simulink model "HealthySubject08062023_Storage"  (R2023a)
settings: Solver=VariableStepAuto  StartTime=0.0  StopTime=3000  RelTol=1e-3
values from neighbouring files (symbols this model uses):
  Cn = 1    [Inhibitory_excitatory_ULInjury_1Hz_08102023.m]    (also in Inhibitory_excitatory_ULInjury_30Hz_08102023.m; InitialExcitatoryInhibitoryNeurons_Healthy08062023.m; InitialExcitatoryInhibitoryULInjured_08102023_DSD.m)
  EK = -84*1    (= -84)    [Inhibitory_excitatory_ULInjury_1Hz_08102023.m]    (also in Inhibitory_excitatory_ULInjury_30Hz_08102023.m; InitialExcitatoryInhibitoryNeurons_Healthy08062023.m; InitialExcitatoryInhibitoryULInjured_08102023_DSD.m)
  EKEx = -90    [Inhibitory_excitatory_ULInjury_1Hz_08102023.m]    (also in Inhibitory_excitatory_ULInjury_30Hz_08102023.m; InitialExcitatoryInhibitoryNeurons_Healthy08062023.m; InitialExcitatoryInhibitoryULInjured_08102023_DSD.m)
  EKIn = -90    [Inhibitory_excitatory_ULInjury_1Hz_08102023.m]    (also in Inhibitory_excitatory_ULInjury_30Hz_08102023.m; InitialExcitatoryInhibitoryNeurons_Healthy08062023.m; InitialExcitatoryInhibitoryULInjured_08102023_DSD.m)
  ELEx = -65    [Inhibitory_excitatory_ULInjury_1Hz_08102023.m]    (also in Inhibitory_excitatory_ULInjury_30Hz_08102023.m; InitialExcitatoryInhibitoryNeurons_Healthy08062023.m; InitialExcitatoryInhibitoryULInjured_08102023_DSD.m)
  ELIn = -65    [Inhibitory_excitatory_ULInjury_1Hz_08102023.m]    (also in Inhibitory_excitatory_ULInjury_30Hz_08102023.m; InitialExcitatoryInhibitoryNeurons_Healthy08062023.m; InitialExcitatoryInhibitoryULInjured_08102023_DSD.m)
  ELk = -83.38*1    (= -83.38)    [Inhibitory_excitatory_ULInjury_1Hz_08102023.m]    (also in Inhibitory_excitatory_ULInjury_30Hz_08102023.m; InitialExcitatoryInhibitoryNeurons_Healthy08062023.m; InitialExcitatoryInhibitoryULInjured_08102023_DSD.m)
  ENa = 50*1    (= 50)    [Inhibitory_excitatory_ULInjury_1Hz_08102023.m]    (also in Inhibitory_excitatory_ULInjury_30Hz_08102023.m; InitialExcitatoryInhibitoryNeurons_Healthy08062023.m; InitialExcitatoryInhibitoryULInjured_08102023_DSD.m)
  ENaEx = 60    [Inhibitory_excitatory_ULInjury_1Hz_08102023.m]    (also in Inhibitory_excitatory_ULInjury_30Hz_08102023.m; InitialExcitatoryInhibitoryNeurons_Healthy08062023.m; InitialExcitatoryInhibitoryULInjured_08102023_DSD.m)
  ENaIn = 55    [Inhibitory_excitatory_ULInjury_1Hz_08102023.m]    (also in Inhibitory_excitatory_ULInjury_30Hz_08102023.m; InitialExcitatoryInhibitoryNeurons_Healthy08062023.m; InitialExcitatoryInhibitoryULInjured_08102023_DSD.m)
  ErestE = -65    [Inhibitory_excitatory_ULInjury_1Hz_08102023.m]    (also in Inhibitory_excitatory_ULInjury_30Hz_08102023.m; InitialExcitatoryInhibitoryNeurons_Healthy08062023.m; InitialExcitatoryInhibitoryULInjured_08102023_DSD.m)
  ErestIn = -64    [Inhibitory_excitatory_ULInjury_1Hz_08102023.m]    (also in Inhibitory_excitatory_ULInjury_30Hz_08102023.m; InitialExcitatoryInhibitoryNeurons_Healthy08062023.m; InitialExcitatoryInhibitoryULInjured_08102023_DSD.m)
  ESynE = -10    [Inhibitory_excitatory_ULInjury_1Hz_08102023.m]    (also in Inhibitory_excitatory_ULInjury_30Hz_08102023.m; InitialExcitatoryInhibitoryNeurons_Healthy08062023.m; InitialExcitatoryInhibitoryULInjured_08102023_DSD.m)
  ESynE2 = -10    [Inhibitory_excitatory_ULInjury_1Hz_08102023.m]    (also in Inhibitory_excitatory_ULInjury_30Hz_08102023.m; InitialExcitatoryInhibitoryNeurons_Healthy08062023.m; InitialExcitatoryInhibitoryULInjured_08102023_DSD.m)
  ESynE3 = -10    [Inhibitory_excitatory_ULInjury_1Hz_08102023.m]    (also in Inhibitory_excitatory_ULInjury_30Hz_08102023.m; InitialExcitatoryInhibitoryNeurons_Healthy08062023.m; InitialExcitatoryInhibitoryULInjured_08102023_DSD.m)
  ESynE4 = -10    [Inhibitory_excitatory_ULInjury_1Hz_08102023.m]    (also in Inhibitory_excitatory_ULInjury_30Hz_08102023.m; InitialExcitatoryInhibitoryNeurons_Healthy08062023.m; InitialExcitatoryInhibitoryULInjured_08102023_DSD.m)
  ESynE5 = -10    [Inhibitory_excitatory_ULInjury_1Hz_08102023.m]    (also in Inhibitory_excitatory_ULInjury_30Hz_08102023.m; InitialExcitatoryInhibitoryNeurons_Healthy08062023.m; InitialExcitatoryInhibitoryULInjured_08102023_DSD.m)
  ESynE610 = -24    [Inhibitory_excitatory_ULInjury_1Hz_08102023.m]    (also in Inhibitory_excitatory_ULInjury_30Hz_08102023.m; InitialExcitatoryInhibitoryNeurons_Healthy08062023.m; InitialExcitatoryInhibitoryULInjured_08102023_DSD.m)
  ESynE6p = -10    [Inhibitory_excitatory_ULInjury_1Hz_08102023.m]    (also in Inhibitory_excitatory_ULInjury_30Hz_08102023.m; InitialExcitatoryInhibitoryNeurons_Healthy08062023.m; InitialExcitatoryInhibitoryULInjured_08102023_DSD.m)
  ESynE7 = -10    [Inhibitory_excitatory_ULInjury_1Hz_08102023.m]    (also in Inhibitory_excitatory_ULInjury_30Hz_08102023.m; InitialExcitatoryInhibitoryNeurons_Healthy08062023.m; InitialExcitatoryInhibitoryULInjured_08102023_DSD.m)
  ESynI = -80    [Inhibitory_excitatory_ULInjury_1Hz_08102023.m]    (also in Inhibitory_excitatory_ULInjury_30Hz_08102023.m; InitialExcitatoryInhibitoryNeurons_Healthy08062023.m; InitialExcitatoryInhibitoryULInjured_08102023_DSD.m)
  ESynI2 = -80    [Inhibitory_excitatory_ULInjury_1Hz_08102023.m]    (also in Inhibitory_excitatory_ULInjury_30Hz_08102023.m; InitialExcitatoryInhibitoryNeurons_Healthy08062023.m; InitialExcitatoryInhibitoryULInjured_08102023_DSD.m)
  ESynI3 = -80    [Inhibitory_excitatory_ULInjury_1Hz_08102023.m]    (also in Inhibitory_excitatory_ULInjury_30Hz_08102023.m; InitialExcitatoryInhibitoryNeurons_Healthy08062023.m; InitialExcitatoryInhibitoryULInjured_08102023_DSD.m)
  ESynI5 = -80    [Inhibitory_excitatory_ULInjury_1Hz_08102023.m]    (also in Inhibitory_excitatory_ULInjury_30Hz_08102023.m; InitialExcitatoryInhibitoryNeurons_Healthy08062023.m; InitialExcitatoryInhibitoryULInjured_08102023_DSD.m)
  ESynI6p = -82    [Inhibitory_excitatory_ULInjury_1Hz_08102023.m]    (also in Inhibitory_excitatory_ULInjury_30Hz_08102023.m; InitialExcitatoryInhibitoryNeurons_Healthy08062023.m; InitialExcitatoryInhibitoryULInjured_08102023_DSD.m)
  Exh0 = ahEx(V0)./(ahEx(V0)+bhEx(V0))    [Inhibitory_excitatory_ULInjury_1Hz_08102023.m]    (also in Inhibitory_excitatory_ULInjury_30Hz_08102023.m; InitialExcitatoryInhibitoryNeurons_Healthy08062023.m; InitialExcitatoryInhibitoryULInjured_08102023_DSD.m)
  Exm0 = amEx(V0)./(amEx(V0)+bmEx(V0))    [Inhibitory_excitatory_ULInjury_1Hz_08102023.m]    (also in Inhibitory_excitatory_ULInjury_30Hz_08102023.m; InitialExcitatoryInhibitoryNeurons_Healthy08062023.m; InitialExcitatoryInhibitoryULInjured_08102023_DSD.m)
  Exn0 = anEx(V0)./(anEx(V0)+bnEx(V0))    [Inhibitory_excitatory_ULInjury_1Hz_08102023.m]    (also in Inhibitory_excitatory_ULInjury_30Hz_08102023.m; InitialExcitatoryInhibitoryNeurons_Healthy08062023.m; InitialExcitatoryInhibitoryULInjured_08102023_DSD.m)
  Ga = 1*Gaxial    (= 0.351233961271)    [Inhibitory_excitatory_ULInjury_1Hz_08102023.m]    (also in Inhibitory_excitatory_ULInjury_30Hz_08102023.m; InitialExcitatoryInhibitoryNeurons_Healthy08062023.m; InitialExcitatoryInhibitoryULInjured_08102023_DSD.m)
  Gaxial = pi*(d^2)/(4*Ro_ax*Internodal_L)*1e7    (= 0.351233961271)    [Inhibitory_excitatory_ULInjury_1Hz_08102023.m]    (also in Inhibitory_excitatory_ULInjury_30Hz_08102023.m; InitialExcitatoryInhibitoryNeurons_Healthy08062023.m; InitialExcitatoryInhibitoryULInjured_08102023_DSD.m)
  gKEx = 100    [Inhibitory_excitatory_ULInjury_1Hz_08102023.m]    (also in Inhibitory_excitatory_ULInjury_30Hz_08102023.m; InitialExcitatoryInhibitoryNeurons_Healthy08062023.m; InitialExcitatoryInhibitoryULInjured_08102023_DSD.m)
  gKIn = 9    [Inhibitory_excitatory_ULInjury_1Hz_08102023.m]    (also in Inhibitory_excitatory_ULInjury_30Hz_08102023.m; InitialExcitatoryInhibitoryNeurons_Healthy08062023.m; InitialExcitatoryInhibitoryULInjured_08102023_DSD.m)
  gKs = 10*0.08/1    (= 0.8)    [Inhibitory_excitatory_ULInjury_1Hz_08102023.m]    (also in Inhibitory_excitatory_ULInjury_30Hz_08102023.m; InitialExcitatoryInhibitoryNeurons_Healthy08062023.m; InitialExcitatoryInhibitoryULInjured_08102023_DSD.m)
  gLEx = 0.1    [Inhibitory_excitatory_ULInjury_1Hz_08102023.m]    (also in Inhibitory_excitatory_ULInjury_30Hz_08102023.m; InitialExcitatoryInhibitoryNeurons_Healthy08062023.m; InitialExcitatoryInhibitoryULInjured_08102023_DSD.m)
  gLIn = 0.1    [Inhibitory_excitatory_ULInjury_1Hz_08102023.m]    (also in Inhibitory_excitatory_ULInjury_30Hz_08102023.m; InitialExcitatoryInhibitoryNeurons_Healthy08062023.m; InitialExcitatoryInhibitoryULInjured_08102023_DSD.m)
  gLk = 10*0.08/1    (= 0.8)    [Inhibitory_excitatory_ULInjury_1Hz_08102023.m]    (also in Inhibitory_excitatory_ULInjury_30Hz_08102023.m; InitialExcitatoryInhibitoryNeurons_Healthy08062023.m; InitialExcitatoryInhibitoryULInjured_08102023_DSD.m)
  gNaEx = 30    [Inhibitory_excitatory_ULInjury_1Hz_08102023.m]    (also in Inhibitory_excitatory_ULInjury_30Hz_08102023.m; InitialExcitatoryInhibitoryNeurons_Healthy08062023.m; InitialExcitatoryInhibitoryULInjured_08102023_DSD.m)
  gNaf = 10*3/1    (= 30)    [Inhibitory_excitatory_ULInjury_1Hz_08102023.m]    (also in Inhibitory_excitatory_ULInjury_30Hz_08102023.m; InitialExcitatoryInhibitoryNeurons_Healthy08062023.m; InitialExcitatoryInhibitoryULInjured_08102023_DSD.m)
  gNaIn = 35    [Inhibitory_excitatory_ULInjury_1Hz_08102023.m]    (also in Inhibitory_excitatory_ULInjury_30Hz_08102023.m; InitialExcitatoryInhibitoryNeurons_Healthy08062023.m; InitialExcitatoryInhibitoryULInjured_08102023_DSD.m)
  gNap = 10*0.005/1    (= 0.05)    [Inhibitory_excitatory_ULInjury_1Hz_08102023.m]    (also in Inhibitory_excitatory_ULInjury_30Hz_08102023.m; InitialExcitatoryInhibitoryNeurons_Healthy08062023.m; InitialExcitatoryInhibitoryULInjured_08102023_DSD.m)
  gSynE = 0.08    [Inhibitory_excitatory_ULInjury_1Hz_08102023.m]    (also in Inhibitory_excitatory_ULInjury_30Hz_08102023.m; InitialExcitatoryInhibitoryNeurons_Healthy08062023.m; InitialExcitatoryInhibitoryULInjured_08102023_DSD.m)
  gSynE2 = 0.08    [Inhibitory_excitatory_ULInjury_1Hz_08102023.m]    (also in Inhibitory_excitatory_ULInjury_30Hz_08102023.m; InitialExcitatoryInhibitoryNeurons_Healthy08062023.m; InitialExcitatoryInhibitoryULInjured_08102023_DSD.m)
  gSynE3 = 0.08    [Inhibitory_excitatory_ULInjury_1Hz_08102023.m]    (also in Inhibitory_excitatory_ULInjury_30Hz_08102023.m; InitialExcitatoryInhibitoryNeurons_Healthy08062023.m; InitialExcitatoryInhibitoryULInjured_08102023_DSD.m)
  gSynE4 = 0.08    [Inhibitory_excitatory_ULInjury_1Hz_08102023.m]    (also in Inhibitory_excitatory_ULInjury_30Hz_08102023.m; InitialExcitatoryInhibitoryNeurons_Healthy08062023.m; InitialExcitatoryInhibitoryULInjured_08102023_DSD.m)
  gSynE5 = 0.08    [Inhibitory_excitatory_ULInjury_1Hz_08102023.m]    (also in Inhibitory_excitatory_ULInjury_30Hz_08102023.m; InitialExcitatoryInhibitoryNeurons_Healthy08062023.m; InitialExcitatoryInhibitoryULInjured_08102023_DSD.m)
  gSynE6 = 0.08    [Inhibitory_excitatory_ULInjury_1Hz_08102023.m]    (also in Inhibitory_excitatory_ULInjury_30Hz_08102023.m; InitialExcitatoryInhibitoryNeurons_Healthy08062023.m; InitialExcitatoryInhibitoryULInjured_08102023_DSD.m)
  gSynE7 = 0.165    [Inhibitory_excitatory_ULInjury_1Hz_08102023.m]    (also in Inhibitory_excitatory_ULInjury_30Hz_08102023.m; InitialExcitatoryInhibitoryNeurons_Healthy08062023.m; InitialExcitatoryInhibitoryULInjured_08102023_DSD.m)
  gSynI = 0.8    [Inhibitory_excitatory_ULInjury_1Hz_08102023.m]    (also in Inhibitory_excitatory_ULInjury_30Hz_08102023.m; InitialExcitatoryInhibitoryNeurons_Healthy08062023.m; InitialExcitatoryInhibitoryULInjured_08102023_DSD.m)
  gSynI2 = 0.12    [Inhibitory_excitatory_ULInjury_1Hz_08102023.m]    (also in Inhibitory_excitatory_ULInjury_30Hz_08102023.m; InitialExcitatoryInhibitoryNeurons_Healthy08062023.m; InitialExcitatoryInhibitoryULInjured_08102023_DSD.m)
  gSynI3 = 0.12    [Inhibitory_excitatory_ULInjury_1Hz_08102023.m]    (also in Inhibitory_excitatory_ULInjury_30Hz_08102023.m; InitialExcitatoryInhibitoryNeurons_Healthy08062023.m; InitialExcitatoryInhibitoryULInjured_08102023_DSD.m)
  gSynI5 = 0.12    [Inhibitory_excitatory_ULInjury_1Hz_08102023.m]    (also in Inhibitory_excitatory_ULInjury_30Hz_08102023.m; InitialExcitatoryInhibitoryNeurons_Healthy08062023.m; InitialExcitatoryInhibitoryULInjured_08102023_DSD.m)
  gSynI6 = 0.12    [Inhibitory_excitatory_ULInjury_1Hz_08102023.m]    (also in Inhibitory_excitatory_ULInjury_30Hz_08102023.m; InitialExcitatoryInhibitoryNeurons_Healthy08062023.m; InitialExcitatoryInhibitoryULInjured_08102023_DSD.m)
  h0 = ah(V0O)./(ah(V0O)+bh(V0O))    [Inhibitory_excitatory_ULInjury_1Hz_08102023.m]    (also in Inhibitory_excitatory_ULInjury_30Hz_08102023.m; InitialExcitatoryInhibitoryNeurons_Healthy08062023.m; InitialExcitatoryInhibitoryULInjured_08102023_DSD.m)
  Inh0 = ahIn(ErestIn)./(ahIn(ErestIn)+bhIn(ErestIn))    [Inhibitory_excitatory_ULInjury_1Hz_08102023.m]    (also in Inhibitory_excitatory_ULInjury_30Hz_08102023.m; InitialExcitatoryInhibitoryNeurons_Healthy08062023.m; InitialExcitatoryInhibitoryULInjured_08102023_DSD.m)
  Inm0 = amIn(ErestIn)./(amIn(ErestIn)+bmIn(ErestIn))    [Inhibitory_excitatory_ULInjury_1Hz_08102023.m]    (also in Inhibitory_excitatory_ULInjury_30Hz_08102023.m; InitialExcitatoryInhibitoryNeurons_Healthy08062023.m; InitialExcitatoryInhibitoryULInjured_08102023_DSD.m)
  Inn0 = anIn(ErestIn)./(anIn(ErestIn)+bnIn(ErestIn))    [Inhibitory_excitatory_ULInjury_1Hz_08102023.m]    (also in Inhibitory_excitatory_ULInjury_30Hz_08102023.m; InitialExcitatoryInhibitoryNeurons_Healthy08062023.m; InitialExcitatoryInhibitoryULInjured_08102023_DSD.m)
  m0 = am(V0O)./(am(V0O)+Bm(V0O))    [Inhibitory_excitatory_ULInjury_1Hz_08102023.m]    (also in Inhibitory_excitatory_ULInjury_30Hz_08102023.m; InitialExcitatoryInhibitoryNeurons_Healthy08062023.m; InitialExcitatoryInhibitoryULInjured_08102023_DSD.m)
  mNap0 = amNap(V0)./(amNap(V0O)+bmNap(V0O))    [Inhibitory_excitatory_ULInjury_1Hz_08102023.m]    (also in Inhibitory_excitatory_ULInjury_30Hz_08102023.m; InitialExcitatoryInhibitoryNeurons_Healthy08062023.m; InitialExcitatoryInhibitoryULInjured_08102023_DSD.m)
  Ro_e = 500    [Inhibitory_excitatory_ULInjury_1Hz_08102023.m]    (also in Inhibitory_excitatory_ULInjury_30Hz_08102023.m; InitialExcitatoryInhibitoryNeurons_Healthy08062023.m; InitialExcitatoryInhibitoryULInjured_08102023_DSD.m)
  s0 = as(V0O)./(as(V0O)+bs(V0O))    [Inhibitory_excitatory_ULInjury_1Hz_08102023.m]    (also in Inhibitory_excitatory_ULInjury_30Hz_08102023.m; InitialExcitatoryInhibitoryNeurons_Healthy08062023.m; InitialExcitatoryInhibitoryULInjured_08102023_DSD.m)
  TawIExt = 30    [Inhibitory_excitatory_ULInjury_1Hz_08102023.m]    (also in Inhibitory_excitatory_ULInjury_30Hz_08102023.m; InitialExcitatoryInhibitoryNeurons_Healthy08062023.m = 200; InitialExcitatoryInhibitoryULInjured_08102023_DSD.m = 200)
  TawIExtE = 30    [Inhibitory_excitatory_ULInjury_1Hz_08102023.m]    (also in Inhibitory_excitatory_ULInjury_30Hz_08102023.m; InitialExcitatoryInhibitoryNeurons_Healthy08062023.m = 1; InitialExcitatoryInhibitoryULInjured_08102023_DSD.m = 10)
  TawSynE = 5    [Inhibitory_excitatory_ULInjury_1Hz_08102023.m]    (also in Inhibitory_excitatory_ULInjury_30Hz_08102023.m; InitialExcitatoryInhibitoryNeurons_Healthy08062023.m; InitialExcitatoryInhibitoryULInjured_08102023_DSD.m)
  TawSynE10 = 5    [Inhibitory_excitatory_ULInjury_1Hz_08102023.m]    (also in Inhibitory_excitatory_ULInjury_30Hz_08102023.m; InitialExcitatoryInhibitoryNeurons_Healthy08062023.m; InitialExcitatoryInhibitoryULInjured_08102023_DSD.m = 3)
  TawSynE2 = 11    [Inhibitory_excitatory_ULInjury_1Hz_08102023.m]    (also in Inhibitory_excitatory_ULInjury_30Hz_08102023.m; InitialExcitatoryInhibitoryNeurons_Healthy08062023.m = 12; InitialExcitatoryInhibitoryULInjured_08102023_DSD.m = 5)
  TawSynE3 = 10    [Inhibitory_excitatory_ULInjury_1Hz_08102023.m]    (also in Inhibitory_excitatory_ULInjury_30Hz_08102023.m; InitialExcitatoryInhibitoryNeurons_Healthy08062023.m = 18; InitialExcitatoryInhibitoryULInjured_08102023_DSD.m = 8)
  TawSynE4 = 6    [Inhibitory_excitatory_ULInjury_1Hz_08102023.m]    (also in Inhibitory_excitatory_ULInjury_30Hz_08102023.m; InitialExcitatoryInhibitoryNeurons_Healthy08062023.m; InitialExcitatoryInhibitoryULInjured_08102023_DSD.m)
  TawSynE41 = 14    [Inhibitory_excitatory_ULInjury_1Hz_08102023.m]    (also in Inhibitory_excitatory_ULInjury_30Hz_08102023.m; InitialExcitatoryInhibitoryNeurons_Healthy08062023.m = 15; InitialExcitatoryInhibitoryULInjured_08102023_DSD.m = 6)
  TawSynE5 = 6    [Inhibitory_excitatory_ULInjury_1Hz_08102023.m]    (also in Inhibitory_excitatory_ULInjury_30Hz_08102023.m; InitialExcitatoryInhibitoryNeurons_Healthy08062023.m; InitialExcitatoryInhibitoryULInjured_08102023_DSD.m)
  TawSynE6 = 3    [Inhibitory_excitatory_ULInjury_1Hz_08102023.m]    (also in Inhibitory_excitatory_ULInjury_30Hz_08102023.m; InitialExcitatoryInhibitoryNeurons_Healthy08062023.m; InitialExcitatoryInhibitoryULInjured_08102023_DSD.m)
  TawSynE66E = 5    [Inhibitory_excitatory_ULInjury_1Hz_08102023.m]    (also in Inhibitory_excitatory_ULInjury_30Hz_08102023.m; InitialExcitatoryInhibitoryNeurons_Healthy08062023.m; InitialExcitatoryInhibitoryULInjured_08102023_DSD.m)
  TawSynE7 = 0.05    [Inhibitory_excitatory_ULInjury_1Hz_08102023.m]    (also in Inhibitory_excitatory_ULInjury_30Hz_08102023.m; InitialExcitatoryInhibitoryNeurons_Healthy08062023.m; InitialExcitatoryInhibitoryULInjured_08102023_DSD.m)
  TawSynI = 5    [Inhibitory_excitatory_ULInjury_1Hz_08102023.m]    (also in Inhibitory_excitatory_ULInjury_30Hz_08102023.m; InitialExcitatoryInhibitoryNeurons_Healthy08062023.m; InitialExcitatoryInhibitoryULInjured_08102023_DSD.m)
  TawSynI2 = 1    [Inhibitory_excitatory_ULInjury_1Hz_08102023.m]    (also in Inhibitory_excitatory_ULInjury_30Hz_08102023.m; InitialExcitatoryInhibitoryNeurons_Healthy08062023.m; InitialExcitatoryInhibitoryULInjured_08102023_DSD.m = 2)
  TawSynI3 = 30    [Inhibitory_excitatory_ULInjury_1Hz_08102023.m]    (also in Inhibitory_excitatory_ULInjury_30Hz_08102023.m; InitialExcitatoryInhibitoryNeurons_Healthy08062023.m = 35; InitialExcitatoryInhibitoryULInjured_08102023_DSD.m)
  TawSynI5 = 4    [Inhibitory_excitatory_ULInjury_1Hz_08102023.m]    (also in Inhibitory_excitatory_ULInjury_30Hz_08102023.m; InitialExcitatoryInhibitoryNeurons_Healthy08062023.m = 1; InitialExcitatoryInhibitoryULInjured_08102023_DSD.m = 1)
  TawSynI6 = 3    [Inhibitory_excitatory_ULInjury_1Hz_08102023.m]    (also in Inhibitory_excitatory_ULInjury_30Hz_08102023.m; InitialExcitatoryInhibitoryNeurons_Healthy08062023.m; InitialExcitatoryInhibitoryULInjured_08102023_DSD.m)
  TawSynI7 = 0.01    [Inhibitory_excitatory_ULInjury_1Hz_08102023.m]    (also in Inhibitory_excitatory_ULInjury_30Hz_08102023.m; InitialExcitatoryInhibitoryNeurons_Healthy08062023.m; InitialExcitatoryInhibitoryULInjured_08102023_DSD.m)
  V0 = -65    [Inhibitory_excitatory_ULInjury_1Hz_08102023.m]    (also in Inhibitory_excitatory_ULInjury_30Hz_08102023.m; InitialExcitatoryInhibitoryNeurons_Healthy08062023.m; InitialExcitatoryInhibitoryULInjured_08102023_DSD.m)
  V0In = -64    [Inhibitory_excitatory_ULInjury_1Hz_08102023.m]    (also in Inhibitory_excitatory_ULInjury_30Hz_08102023.m; InitialExcitatoryInhibitoryNeurons_Healthy08062023.m; InitialExcitatoryInhibitoryULInjured_08102023_DSD.m)
  w10 = 0.035    [Inhibitory_excitatory_ULInjury_1Hz_08102023.m]    (also in Inhibitory_excitatory_ULInjury_30Hz_08102023.m; InitialExcitatoryInhibitoryNeurons_Healthy08062023.m)
  w12 = -0.2    [Inhibitory_excitatory_ULInjury_1Hz_08102023.m]    (also in Inhibitory_excitatory_ULInjury_30Hz_08102023.m; InitialExcitatoryInhibitoryNeurons_Healthy08062023.m = -0.28; InitialExcitatoryInhibitoryULInjured_08102023_DSD.m = -0.35)
  w14 = 0.05    [Inhibitory_excitatory_ULInjury_1Hz_08102023.m]    (also in Inhibitory_excitatory_ULInjury_30Hz_08102023.m; InitialExcitatoryInhibitoryNeurons_Healthy08062023.m = 0.09; InitialExcitatoryInhibitoryULInjured_08102023_DSD.m = 0.09)
  w15 = -0.45    [Inhibitory_excitatory_ULInjury_1Hz_08102023.m]    (also in Inhibitory_excitatory_ULInjury_30Hz_08102023.m = -0.07; InitialExcitatoryInhibitoryNeurons_Healthy08062023.m = -0.4; InitialExcitatoryInhibitoryULInjured_08102023_DSD.m = -0.4)
  w17 = -0.25    [Inhibitory_excitatory_ULInjury_1Hz_08102023.m]    (also in Inhibitory_excitatory_ULInjury_30Hz_08102023.m; InitialExcitatoryInhibitoryNeurons_Healthy08062023.m; InitialExcitatoryInhibitoryULInjured_08102023_DSD.m)
  w26 = 0.2    [Inhibitory_excitatory_ULInjury_1Hz_08102023.m]    (also in Inhibitory_excitatory_ULInjury_30Hz_08102023.m = 0.25; InitialExcitatoryInhibitoryNeurons_Healthy08062023.m = 0.05; InitialExcitatoryInhibitoryULInjured_08102023_DSD.m = 0.05)
  w28 = 0.165    [Inhibitory_excitatory_ULInjury_1Hz_08102023.m]    (also in Inhibitory_excitatory_ULInjury_30Hz_08102023.m; InitialExcitatoryInhibitoryNeurons_Healthy08062023.m = 0.13; InitialExcitatoryInhibitoryULInjured_08102023_DSD.m = 0.13)
  w34 = 0.09    [Inhibitory_excitatory_ULInjury_1Hz_08102023.m]    (also in Inhibitory_excitatory_ULInjury_30Hz_08102023.m; InitialExcitatoryInhibitoryNeurons_Healthy08062023.m = 0.03; InitialExcitatoryInhibitoryULInjured_08102023_DSD.m = 0.06)
  w63 = -0.12    [Inhibitory_excitatory_ULInjury_1Hz_08102023.m]    (also in Inhibitory_excitatory_ULInjury_30Hz_08102023.m; InitialExcitatoryInhibitoryNeurons_Healthy08062023.m = -0.08; InitialExcitatoryInhibitoryULInjured_08102023_DSD.m = -0.27)
  w66E = 0.2    [Inhibitory_excitatory_ULInjury_1Hz_08102023.m]    (also in Inhibitory_excitatory_ULInjury_30Hz_08102023.m; InitialExcitatoryInhibitoryNeurons_Healthy08062023.m = 0.09; InitialExcitatoryInhibitoryULInjured_08102023_DSD.m = 0.1)
  w67 = -0.4    [Inhibitory_excitatory_ULInjury_1Hz_08102023.m]    (also in Inhibitory_excitatory_ULInjury_30Hz_08102023.m; InitialExcitatoryInhibitoryNeurons_Healthy08062023.m = -0.55; InitialExcitatoryInhibitoryULInjured_08102023_DSD.m = -0.55)
  w68 = 0.35    [Inhibitory_excitatory_ULInjury_1Hz_08102023.m]    (also in Inhibitory_excitatory_ULInjury_30Hz_08102023.m; InitialExcitatoryInhibitoryNeurons_Healthy08062023.m = 0.1; InitialExcitatoryInhibitoryULInjured_08102023_DSD.m = 0.1)
  w71 = 0.25    [Inhibitory_excitatory_ULInjury_1Hz_08102023.m]    (also in Inhibitory_excitatory_ULInjury_30Hz_08102023.m; InitialExcitatoryInhibitoryNeurons_Healthy08062023.m; InitialExcitatoryInhibitoryULInjured_08102023_DSD.m)
  w78 = 0.25    [Inhibitory_excitatory_ULInjury_1Hz_08102023.m]    (also in Inhibitory_excitatory_ULInjury_30Hz_08102023.m; InitialExcitatoryInhibitoryNeurons_Healthy08062023.m; InitialExcitatoryInhibitoryULInjured_08102023_DSD.m)
  w79 = 0.35    [Inhibitory_excitatory_ULInjury_1Hz_08102023.m]    (also in Inhibitory_excitatory_ULInjury_30Hz_08102023.m; InitialExcitatoryInhibitoryNeurons_Healthy08062023.m; InitialExcitatoryInhibitoryULInjured_08102023_DSD.m)
  w83 = 0.2    [Inhibitory_excitatory_ULInjury_1Hz_08102023.m]    (also in Inhibitory_excitatory_ULInjury_30Hz_08102023.m; InitialExcitatoryInhibitoryNeurons_Healthy08062023.m = 0.13; InitialExcitatoryInhibitoryULInjured_08102023_DSD.m = 0.08)
  w85 = 0.1    [Inhibitory_excitatory_ULInjury_1Hz_08102023.m]    (also in Inhibitory_excitatory_ULInjury_30Hz_08102023.m = 0.12; InitialExcitatoryInhibitoryNeurons_Healthy08062023.m = 0.04; InitialExcitatoryInhibitoryULInjured_08102023_DSD.m = 0.05)
  X = nan(node,1)    [Inhibitory_excitatory_ULInjury_1Hz_08102023.m]    (also in Inhibitory_excitatory_ULInjury_30Hz_08102023.m; InitialExcitatoryInhibitoryNeurons_Healthy08062023.m; InitialExcitatoryInhibitoryULInjured_08102023_DSD.m)
  X2 = nan(node2,1)    [Inhibitory_excitatory_ULInjury_1Hz_08102023.m]    (also in Inhibitory_excitatory_ULInjury_30Hz_08102023.m; InitialExcitatoryInhibitoryNeurons_Healthy08062023.m; InitialExcitatoryInhibitoryULInjured_08102023_DSD.m)
  Xelec = Xtotal-Nodal_L*9-Internodal_L*9    (= 0.1152)    [Inhibitory_excitatory_ULInjury_1Hz_08102023.m]    (also in Inhibitory_excitatory_ULInjury_30Hz_08102023.m; InitialExcitatoryInhibitoryNeurons_Healthy08062023.m; InitialExcitatoryInhibitoryULInjured_08102023_DSD.m)
  Xelec2 = 1/(10000)+Nodal_L2*(node2-1)/2+Internodal_L2*(node2-1)/2    (= 0.0001)    [Inhibitory_excitatory_ULInjury_1Hz_08102023.m]    (also in Inhibitory_excitatory_ULInjury_30Hz_08102023.m; InitialExcitatoryInhibitoryNeurons_Healthy08062023.m; InitialExcitatoryInhibitoryULInjured_08102023_DSD.m)
  Y = nan(node,1)    [Inhibitory_excitatory_ULInjury_1Hz_08102023.m]    (also in Inhibitory_excitatory_ULInjury_30Hz_08102023.m; InitialExcitatoryInhibitoryNeurons_Healthy08062023.m; InitialExcitatoryInhibitoryULInjured_08102023_DSD.m)
  Y2 = nan(node2,1)    [Inhibitory_excitatory_ULInjury_1Hz_08102023.m]    (also in Inhibitory_excitatory_ULInjury_30Hz_08102023.m; InitialExcitatoryInhibitoryNeurons_Healthy08062023.m; InitialExcitatoryInhibitoryULInjured_08102023_DSD.m)
  Yelec = 100/10000    (= 0.01)    [Inhibitory_excitatory_ULInjury_1Hz_08102023.m]    (also in Inhibitory_excitatory_ULInjury_30Hz_08102023.m; InitialExcitatoryInhibitoryNeurons_Healthy08062023.m; InitialExcitatoryInhibitoryULInjured_08102023_DSD.m)
  Yelec2 = 500/10000    (= 0.05)    [Inhibitory_excitatory_ULInjury_1Hz_08102023.m]    (also in Inhibitory_excitatory_ULInjury_30Hz_08102023.m; InitialExcitatoryInhibitoryNeurons_Healthy08062023.m; InitialExcitatoryInhibitoryULInjured_08102023_DSD.m)
(part 1 of 13)
settings Model: Creator=mfard  LastModifiedBy=mfard
settings SolverCC: AlgebraicLoopSolver=TrustRegion
settings DebuggingCC: UnconnectedInputMsg=warning  UnconnectedOutputMsg=warning  UnconnectedLineMsg=warning
settings ModelReferenceCC: EnableRefExpFcnMdlSchedulingChecks=on

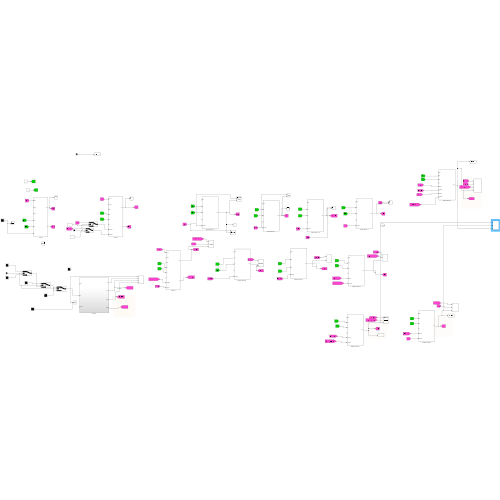
[thumbnail: Simulink's stored preview of the top-level diagram]
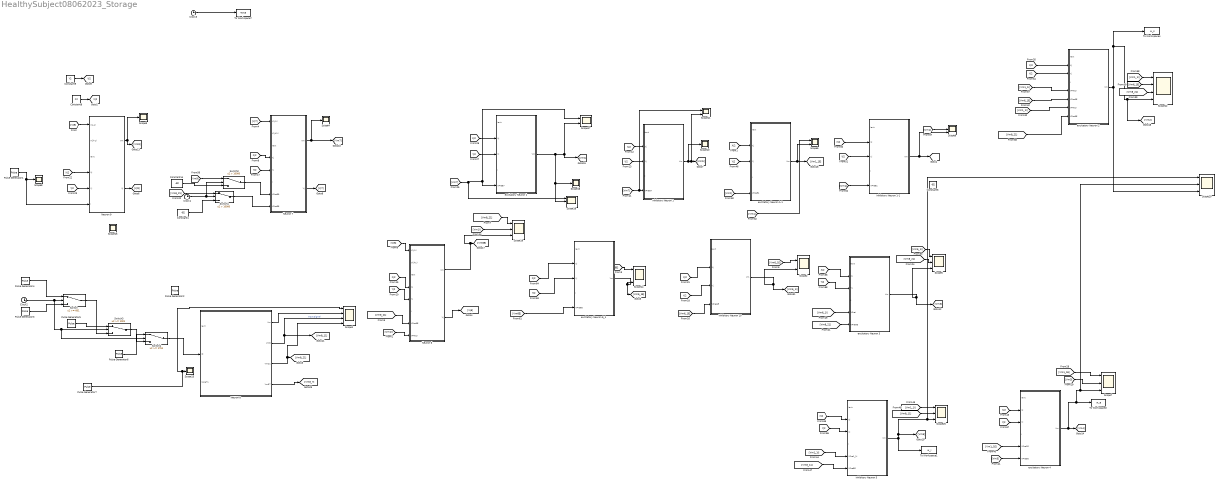
== system HealthySubject08062023_Storage ==
  Clock1 : Clock
  Clock2 : Clock
  Clock3 : Clock
  Constant1 : Constant  Value=-82
  Constant14 : Constant  Value=-82
  Constant6 : Constant  Value=-82
  Constant8 : Constant  Value=X2
  Constant9 : Constant  Value=Y2
  Inhibitory Neuron 1 : Subsystem
      mask init:
      | p=1
  Inhibitory Neuron 1-1 : Subsystem
      mask init:
      | p=1
  Inhibitory Neuron 10 : Subsystem
      mask init:
      | p=1
  Inhibitory Neuron 5 : Subsystem
      mask init:
      | p=1
  Neuron 6 : Subsystem
      mask init:
      | p=1
  Neuron 7 : Subsystem
      mask init:
      | p=1
  Neuron 8 : Subsystem
  Neuron 9 : Subsystem
      mask init:
      | p=1
  Pulse Generator1 : DiscretePulseGenerator  PulseType=Time based  Amplitude=15  Period=10  PulseWidth=30
  Pulse Generator2 : DiscretePulseGenerator  PulseType=Time based  Amplitude=20  Period=20  PulseWidth=5
  Pulse Generator3 : DiscretePulseGenerator  PulseType=Time based  Amplitude=15  Period=150  PulseWidth=5
  Pulse Generator4 : DiscretePulseGenerator  PulseType=Time based  Amplitude=15  Period=100  PulseWidth=5
  Pulse Generator5 : DiscretePulseGenerator  PulseType=Time based  Amplitude=15  Period=75  PulseWidth=5
  Pulse Generator6 : DiscretePulseGenerator  PulseType=Time based  Amplitude=20  Period=24  PulseWidth=5
  Pulse Generator7 : DiscretePulseGenerator  PulseType=Time based  Amplitude=20  Period=20  PulseWidth=5
  Scope1 : Scope  NumInputPorts=4
  Scope{3..4,8,10,13,15..16} (7 alike) : Scope
  Scope{2,6,11,17} (4 alike) : Scope  NumInputPorts=2
  Scope12 : Scope  NumInputPorts=4
  Scope{5,7,9,14,18..20,25} (8 alike) : Scope  NumInputPorts=3
  Switch : Switch  Threshold=601  SaturateOnIntegerOverflow=off  InputSameDT=off
  Switch1 : Switch  Criteria=u2 > Threshold  Threshold=10000  SaturateOnIntegerOverflow=off  InputSameDT=off
  Switch2 : Switch  Criteria=u2 > Threshold  Threshold=10000  SaturateOnIntegerOverflow=off  InputSameDT=off
  Switch3 : Switch  Threshold=1001  SaturateOnIntegerOverflow=off  InputSameDT=off
  Switch4 : Switch  Threshold=1751  SaturateOnIntegerOverflow=off  InputSameDT=off
  To Workspace1 : ToWorkspace  VariableName=w_i  SampleTime=-1
  To Workspace2 : ToWorkspace  VariableName=w_e  SampleTime=-1
  To Workspace4 : ToWorkspace  VariableName=w_s  SampleTime=-1
  To Workspace7 : ToWorkspace  VariableName=Time  SampleTime=-1
  excitatory Neuron 1 : Subsystem
      mask init:
      | p=1
  excitatory Neuron 1-1 : Subsystem
      mask init:
      | p=1
  excitatory Neuron 2 : Subsystem
      mask init:
      | p=1
  excitatory Neuron 3 : Subsystem
      mask init:
      | p=1
  excitatory Neuron 4 : Subsystem
      mask init:
      | p=1
  excitatory Neuron 6_1 : Subsystem
      mask init:
      | p=1
  tag scope: Xj2=global, Yj2=global
  wires:
  [Vm1] -> excitatory Neuron 1-1/5(VPreE1)
  [Vm1] -> Inhibitory Neuron 1-1/5(VPreE1)
  [Vm6E] -> excitatory Neuron 6_1/5(VPre6E)
  [Vm7] -> Scope11/1, Inhibitory Neuron 1/5(VPreE7)
  [Vj6] -> Neuron 6/1(V(j-1))
  Neuron 7/1(Vm) -> Scope4/1, [Vm7]
  [Xj2] -> Neuron 6/4(Xj)
  [Xj2] -> Inhibitory Neuron 1/2(Xj)
  excitatory Neuron 1/1(Vm) -> Scope17/2, [Vm1], Scope16/1, Scope18/2
  Switch/1 -> Switch3/3
  [Vm8_21] -> Switch1/1
  [Yj2] -> excitatory Neuron 1/3(Yj)
  Neuron 9/1(Vm) -> [Vm9], Scope3/1
  [Vm1I] -> Neuron 6/8(VPre1I)
  Switch3/1 -> Switch4/3
  [Xj2] -> excitatory Neuron 6_1/2(Xj)
  [Vm1I] -> Scope19/2
  [Xj2] -> Neuron 9/4(Xj)
  Pulse Generator1/1 -> Neuron 9/6("I "), Scope8/1
  [Yj2] -> Inhibitory Neuron 1-1/3(Yj)
  [Yj2] -> Neuron 9/5(Yj)
  Constant1/1 -> Switch1/3
  [Xj2] -> Inhibitory Neuron 1-1/2(Xj)
  [Yj2] -> Neuron 7/5(Yj)
  Constant8/1 -> [Xj2]
  Inhibitory Neuron 1/1(Vm) -> Scope10/1, Scope11/2, [Vm1I]
  [Yj2] -> Inhibitory Neuron 1/3(Yj)
  [Vj7] -> Neuron 7/1(V(j-1))
  [Yj2] -> Inhibitory Neuron 10/3(Yj)
  Switch1/1 -> Neuron 7/8(VPreE8)
  Inhibitory Neuron 1-1/1(Vm) -> Scope9/3, [Vm1_1I]
  Neuron 9/2(Vj) -> [Vj9]
  Neuron 8/4(Vm87) -> [Vm8_7]
  Switch2/1 -> Neuron 7/7("VPreE9 ")
  [Vm1] -> Scope9/2
  [Vm1] -> Scope6/1
  Neuron 6/1(Vm) -> Scope19/3, [Vm6E]
  [Vm7] -> Scope17/1, excitatory Neuron 1/5(VPreE7), Scope18/1
  Inhibitory Neuron 10/1(Vm) -> Scope2/2, [Vm6_1I]
  Clock2/1 -> Switch4/2, Switch3/2, Switch/2
  Constant9/1 -> [Yj2]
  Pulse Generator7/1 -> Scope1/1, Scope13/1
  [Xj2] -> excitatory Neuron 1/2(Xj)
  Pulse Generator3/1 -> Switch/3
  [Vm6_1E] -> Inhibitory Neuron 10/4(VPre6E)
  Pulse Generator5/1 -> Switch3/1
  [Vj9] -> Neuron 9/1(V(j-1))
  [Yj2] -> excitatory Neuron 6_1/3(Yj)
  Pulse Generator4/1 -> Switch/1
  [Vm6E] -> Scope14/1
  excitatory Neuron 1-1/1(Vm) -> Scope6/2, [Vm1_1E]
  Neuron 8/2(Vm5) -> Scope1/3, [Vm8_11]  "Input Signal"
  [Vm8_21] -> Neuron 6/7(VPre8E)
  Neuron 8/1(Vm) -> Scope1/2
  Pulse Generator6/1 -> Switch4/1
  [Xj2] -> excitatory Neuron 1-1/2(Xj)
  excitatory Neuron 6_1/1(Vm) -> Scope14/3, [Vm6_1E]
  Clock1/1 -> Switch2/2, Switch1/2
  [Xj2] -> Inhibitory Neuron 10/2(Xj)
  Neuron 8/3(Vm21) -> Scope1/4, [Vm8_21]
  [Yj2] -> Neuron 6/5(Yj)
  Constant14/1 -> Switch2/3
  [Vm9] -> Switch2/1
  [Vm6_1E] -> Scope2/1
  [Xj2] -> Neuron 7/4(Xj)
  Clock3/1 -> To Workspace7/1
  [Vm8_21] -> Scope19/1
  Neuron 7/2(Vj) -> [Vj7]
  [Yj2] -> excitatory Neuron 1-1/3(Yj)
  Neuron 6/2(Vj) -> [Vj6]
  [Vm8_21] -> excitatory Neuron 3/6(VPre8E)
  [Vm8_21] -> Scope5/2
  excitatory Neuron 3/1(Vm) -> Scope5/3, [Vm3]
  [Vm6_1I] -> excitatory Neuron 3/5("VPreI ")
  [Yj2] -> excitatory Neuron 3/3(Yj)
  [Xj2] -> excitatory Neuron 3/2(Xj)
  [Vm6_1I] -> Scope5/1
  Inhibitory Neuron 5/1(Vm) -> Scope20/1, Scope25/3, [Vm5], To Workspace1/1
  excitatory Neuron 4/1(Vm) -> Scope20/2, Scope7/3, To Workspace2/1, [Vm4]
  [Vm1_1E] -> excitatory Neuron 4/5("VPre1E ")
  [Yj2] -> Inhibitory Neuron 5/3(Yj)
  [Vm1_1I] -> Inhibitory Neuron 5/5("VPre1_1I ")
  [Vm1_1I] -> Scope25/1
  [Vm3] -> Scope7/2
  [Yj2] -> excitatory Neuron 4/3(Yj)
  [Xj2] -> excitatory Neuron 4/2(Xj)
  [Xj2] -> Inhibitory Neuron 5/2(Xj)
  [Vm8_11] -> Scope25/2
  [Vm3] -> excitatory Neuron 4/6(VPre3E)
  [Vm8_11] -> Inhibitory Neuron 5/6(VPre8E)
  [Vm1_1E] -> Scope7/1
  excitatory Neuron 2/1(Vm) -> To Workspace4/1, [Vm2], Scope12/4, Scope20/3
  [Vm8_21] -> excitatory Neuron 2/8(VPre8E)
  [Vm1_1I] -> Scope12/1
  [Vm8_21] -> Scope12/3
  [Vm1_1I] -> excitatory Neuron 2/7(VPre1I)
  [Vm1_1I] -> excitatory Neuron 2/5("VPre1I ")
  [Vm6_1E] -> Scope12/2
  [Vm6_1E] -> excitatory Neuron 2/6(VPre6E)
  [Xj2] -> excitatory Neuron 2/2(Xj)
  [Yj2] -> excitatory Neuron 2/3(Yj)
  Switch4/1 -> Neuron 8/2(I0)

== system HealthySubject08062023_Storage/Inhibitory Neuron 1 ==
  Iext : Inport
  Xj : Inport  Port=2
  Yj : Inport  Port=3
  "I " : Inport  Port=4
  VPreE7 : Inport  Port=5
  Add : Sum  Inputs=+---+-
  Add1 : Sum  Inputs=+-
  Constant2 : Constant  Value=ENaIn
  Divide : Product  Inputs=**
  Gain : Gain  Gain=1/Cn
  Integrator : Integrator  InitialCondition=V0In
  Ks : Subsystem
  Lk : Subsystem
  Naf : Subsystem
  Nap1 : Subsystem
  Scope{1..3,5} (4 alike) : Scope
  Selector : Selector  InputPortWidth=1  IndexOptions=Index vector (dialog)  Indices=p  OutputSizes=1
  Selector1 : Selector  InputPortWidth=1  IndexOptions=Index vector (dialog)  Indices=p  OutputSizes=1
  Subsystem : Subsystem
  Transfer Fcn1 : TransferFcn  Denominator=[TawIExt 1]
  Vm : Outport  VectorParamsAs1DForOutWhenUnconnected=off
  wires:
  Divide/1 -> Add/1
  Ks/1(IKs) -> Add/3
  Naf/1("INaf ") -> Add/2
  Add/1 -> Scope3/1, Gain/1
  Transfer Fcn1/1 -> Scope1/1, Divide/2
  Gain/1 -> Integrator/1
  Subsystem/1(ku) -> Transfer Fcn1/1
  Xj/1 -> Selector/1
  Iext/1 -> Subsystem/1(Iext)
  Selector/1 -> Subsystem/2(Xj)
  Selector1/1 -> Subsystem/3(Yj)
  Yj/1 -> Selector1/1
  Add1/1 -> Divide/1
  Constant2/1 -> Add1/1
  "I "/1 -> Add/5
  Lk/1(ILk) -> Add/4, Scope5/1
  Nap1/1("ISynE ") -> Add/6
  Integrator/1 -> Vm/1, Nap1/1(V), Add1/2, Naf/1(Vm), Ks/1(Vm), Lk/1(Vm)
  VPreE7/1 -> Nap1/2(Pre)

== system HealthySubject08062023_Storage/Inhibitory Neuron 1-1 ==
  Iext : Inport
  Xj : Inport  Port=2
  Yj : Inport  Port=3
  "I " : Inport  Port=4
  VPreE1 : Inport  Port=5
  Add : Sum  Inputs=+---+-
  Add1 : Sum  Inputs=+-
  Constant2 : Constant  Value=ENaIn
  Divide : Product  Inputs=**
  Gain : Gain  Gain=1/Cn
  Integrator : Integrator  InitialCondition=V0In
  Ks : Subsystem
  Lk : Subsystem
  Naf : Subsystem
  Nap1 : Subsystem
  Scope{1..3,5} (4 alike) : Scope
  Selector : Selector  InputPortWidth=1  IndexOptions=Index vector (dialog)  Indices=p  OutputSizes=1
  Selector1 : Selector  InputPortWidth=1  IndexOptions=Index vector (dialog)  Indices=p  OutputSizes=1
  Subsystem : Subsystem
  Transfer Fcn1 : TransferFcn  Denominator=[TawIExt 1]
  Vm : Outport  VectorParamsAs1DForOutWhenUnconnected=off
  wires:
  Divide/1 -> Add/1
  Ks/1(IKs) -> Add/3
  Naf/1("INaf ") -> Add/2
  Add/1 -> Scope3/1, Gain/1
  Transfer Fcn1/1 -> Scope1/1, Divide/2
  Gain/1 -> Integrator/1
  Subsystem/1(ku) -> Transfer Fcn1/1
  Xj/1 -> Selector/1
  Iext/1 -> Subsystem/1(Iext)
  Selector/1 -> Subsystem/2(Xj)
  Selector1/1 -> Subsystem/3(Yj)
  Yj/1 -> Selector1/1
  Add1/1 -> Divide/1
  Constant2/1 -> Add1/1
  Integrator/1 -> Nap1/1(V), Vm/1, Add1/2, Naf/1(Vm), Ks/1(Vm), Lk/1(Vm)
  "I "/1 -> Add/5
  Lk/1(ILk) -> Add/4, Scope5/1
  Nap1/1("ISynE ") -> Add/6
  VPreE1/1 -> Nap1/2(Pre)

== system HealthySubject08062023_Storage/Inhibitory Neuron 10 ==
  Iext : Inport
  Xj : Inport  Port=2
  Yj : Inport  Port=3
  VPre6E : Inport  Port=4
  Add : Sum  Inputs=+---+--
  Add1 : Sum  Inputs=+-
  Constant2 : Constant  Value=ENaIn
  Divide : Product  Inputs=**
  Gain : Gain  Gain=1/Cn
  Integrator : Integrator  InitialCondition=V0In
  Ks : Subsystem
  Lk : Subsystem
  Naf : Subsystem
  Nap2 : Subsystem
  Scope{1..6} (6 alike) : Scope
  Selector : Selector  InputPortWidth=1  IndexOptions=Index vector (dialog)  Indices=p  OutputSizes=1
  Selector1 : Selector  InputPortWidth=1  IndexOptions=Index vector (dialog)  Indices=p  OutputSizes=1
  Subsystem : Subsystem
  Transfer Fcn1 : TransferFcn  Denominator=[TawIExt 1]
  Vm : Outport  VectorParamsAs1DForOutWhenUnconnected=off
  wires:
  Divide/1 -> Add/1
  Naf/1("INaf ") -> Scope4/1, Add/2
  Add/1 -> Scope3/1, Gain/1
  Transfer Fcn1/1 -> Scope1/1, Divide/2
  Gain/1 -> Integrator/1
  Subsystem/1(ku) -> Transfer Fcn1/1
  Xj/1 -> Selector/1
  Iext/1 -> Subsystem/1(Iext)
  Selector/1 -> Subsystem/2(Xj)
  Selector1/1 -> Subsystem/3(Yj)
  Yj/1 -> Selector1/1
  Add1/1 -> Divide/1
  Constant2/1 -> Add1/1
  Nap2/1("ISynE ") -> Scope2/1, Add/6
  VPre6E/1 -> Nap2/2(Pre)
  Integrator/1 -> Vm/1, Nap2/1(V), Add1/2, Naf/1(Vm), Ks/1(Vm), Lk/1(Vm)
  Lk/1(ILk) -> Scope5/1, Add/4
  Ks/1(IKs) -> Scope6/1, Add/3

== system HealthySubject08062023_Storage/Inhibitory Neuron 5 ==
  Iext : Inport
  Xj : Inport  Port=2
  Yj : Inport  Port=3
  "I " : Inport  Port=4
  "VPre1_1I " : Inport  Port=5
  VPre8E : Inport  Port=6
  Add : Sum  Inputs=+---+---
  Add1 : Sum  Inputs=+-
  Constant2 : Constant  Value=ENaIn
  Divide : Product  Inputs=**
  Gain : Gain  Gain=1/Cn
  Integrator : Integrator  InitialCondition=V0In
  Ks : Subsystem
  Lk : Subsystem
  Naf : Subsystem
  Nap1 : Subsystem
  Nap2 : Subsystem
  Nap3 : Subsystem
  Scope{1..3,5} (4 alike) : Scope
  Selector : Selector  InputPortWidth=1  IndexOptions=Index vector (dialog)  Indices=p  OutputSizes=1
  Selector1 : Selector  InputPortWidth=1  IndexOptions=Index vector (dialog)  Indices=p  OutputSizes=1
  Subsystem : Subsystem
  Transfer Fcn1 : TransferFcn  Denominator=[TawIExt 1]
  Vm : Outport  VectorParamsAs1DForOutWhenUnconnected=off
  wires:
  Divide/1 -> Add/1
  Ks/1(IKs) -> Add/3
  Naf/1("INaf ") -> Add/2
  Add/1 -> Scope3/1, Gain/1
  Transfer Fcn1/1 -> Scope1/1, Divide/2
  Gain/1 -> Integrator/1
  Subsystem/1(ku) -> Transfer Fcn1/1
  Xj/1 -> Selector/1
  Iext/1 -> Subsystem/1(Iext)
  Selector/1 -> Subsystem/2(Xj)
  Selector1/1 -> Subsystem/3(Yj)
  Yj/1 -> Selector1/1
  Add1/1 -> Divide/1
  Constant2/1 -> Add1/1
  "I "/1 -> Add/5
  Lk/1(ILk) -> Scope5/1, Add/4
  Integrator/1 -> Nap2/1(V), Vm/1, Nap3/1(V), Nap1/1(V), Add1/2, Naf/1(Vm), Ks/1(Vm), Lk/1(Vm)
  "VPre1_1I "/1 -> Nap1/2(Pre), Nap2/2(Pre)
  VPre8E/1 -> Nap3/2(Pre)
  Nap1/1("ISynE ") -> Add/6
  Nap2/1("ISynI ") -> Add/7
  Nap3/1("ISynE ") -> Add/8

== system HealthySubject08062023_Storage/Neuron 6 ==
  V(j-1) : Inport
  "V(j+1) " : Inport  Port=2
  Iext : Inport  Port=3
  Xj : Inport  Port=4
  Yj : Inport  Port=5
  "I " : Inport  Port=6
  VPre8E : Inport  Port=7
  VPre1I : Inport  Port=8
  Add : Sum  Inputs=+---++-----
  Add1 : Sum  Inputs=+-+
  Constant : Constant  Value=Gaxial
  Divide : Product  Inputs=**
  Gain : Gain  Gain=1/Cn
  Gain1 : Gain  Gain=2
  Integrator : Integrator  InitialCondition=-65
  Ks : Subsystem
  Lk : Subsystem
  Naf : Subsystem
  Nap : Subsystem
  Nap1 : Subsystem
  Nap2 : Subsystem
  Scope{,1..3} (4 alike) : Scope
  Selector : Selector  InputPortWidth=1  IndexOptions=Index vector (dialog)  Indices=p  OutputSizes=1
  Selector1 : Selector  InputPortWidth=1  IndexOptions=Index vector (dialog)  Indices=p  OutputSizes=1
  Subsystem : Subsystem
  Vm : Outport  VectorParamsAs1DForOutWhenUnconnected=off
  Vj : Outport  Port=2  VectorParamsAs1DForOutWhenUnconnected=off
  wires:
  Divide/1 -> Scope/1, Add/1
  Ks/1(IKs) -> Add/3
  Naf/1("INaf ") -> Add/2
  Add/1 -> Scope3/1, Gain/1
  Lk/1(ILk) -> Add/4
  Add1/1 -> Divide/2
  Gain/1 -> Integrator/1
  Gain1/1 -> Add1/2
  Subsystem/1(Vj) -> Gain1/1, Vj/1
  V(j-1)/1 -> Add1/1
  "V(j+1) "/1 -> Add1/3
  Xj/1 -> Selector/1
  Iext/1 -> Subsystem/1(Iext)
  Selector/1 -> Subsystem/2(Xj)
  Selector1/1 -> Subsystem/3(Yj)
  Yj/1 -> Selector1/1
  "I "/1 -> Add/5
  Constant/1 -> Divide/1
  Nap/1("INap ") -> Add/7
  Nap2/1("ISynI ") -> Add/9, Scope2/1
  Nap1/1("ISynE ") -> Scope1/1, Add/8
  ? -> Add/10
  ? -> Add/11
  ? -> Add/6
  VPre1I/1 -> Nap2/2(Pre)
  VPre8E/1 -> Nap1/2(Pre)
  Integrator/1 -> Vm/1, Nap1/1(V), Nap/1(Vm), Lk/1(Vm), Ks/1(Vm), Naf/1(Vm), Nap2/1(V)

== system HealthySubject08062023_Storage/Neuron 7 ==
  V(j-1) : Inport
  "V(j+1) " : Inport  Port=2
  Iext : Inport  Port=3
  Xj : Inport  Port=4
  Yj : Inport  Port=5
  "I " : Inport  Port=6
  "VPreE9 " : Inport  Port=7
  VPreE8 : Inport  Port=8
  Add : Sum  Inputs=+---++-----
  Add1 : Sum  Inputs=+-+
  Constant : Constant  Value=Gaxial
  Divide : Product  Inputs=**
  Gain : Gain  Gain=1/Cn
  Gain1 : Gain  Gain=2
  Integrator : Integrator  InitialCondition=-82
  Ks : Subsystem
  Lk : Subsystem
  Naf : Subsystem
  Nap : Subsystem
  Nap2 : Subsystem
  Nap3 : Subsystem
  Scope{,1..3} (4 alike) : Scope
  Selector : Selector  InputPortWidth=1  IndexOptions=Index vector (dialog)  Indices=p  OutputSizes=1
  Selector1 : Selector  InputPortWidth=1  IndexOptions=Index vector (dialog)  Indices=p  OutputSizes=1
  Subsystem : Subsystem
  Vm : Outport  VectorParamsAs1DForOutWhenUnconnected=off
  Vj : Outport  Port=2  VectorParamsAs1DForOutWhenUnconnected=off
  wires:
  Divide/1 -> Scope/1, Add/1
  Ks/1(IKs) -> Add/3
  Naf/1("INaf ") -> Add/2
  Add/1 -> Scope3/1, Gain/1
  Lk/1(ILk) -> Add/4
  Add1/1 -> Divide/2
  Gain/1 -> Integrator/1
  Gain1/1 -> Add1/2
  Subsystem/1(Vj) -> Gain1/1, Vj/1
  V(j-1)/1 -> Add1/1
  "V(j+1) "/1 -> Add1/3
  Xj/1 -> Selector/1
  Iext/1 -> Subsystem/1(Iext)
  Selector/1 -> Subsystem/2(Xj)
  Selector1/1 -> Subsystem/3(Yj)
  Yj/1 -> Selector1/1
  "I "/1 -> Add/5
  Constant/1 -> Divide/1
  Nap/1("INap ") -> Add/7
  Nap2/1("ISynE ") -> Scope1/1, Add/8
  ? -> Add/10
  ? -> Add/11
  ? -> Add/6
  Integrator/1 -> Vm/1, Nap3/1(V), Nap2/1(V), Nap/1(Vm), Lk/1(Vm), Ks/1(Vm), Naf/1(Vm)
  VPreE8/1 -> Nap2/2(Pre)
  "VPreE9 "/1 -> Nap3/2(Pre)
  Nap3/1("ISynI ") -> Add/9

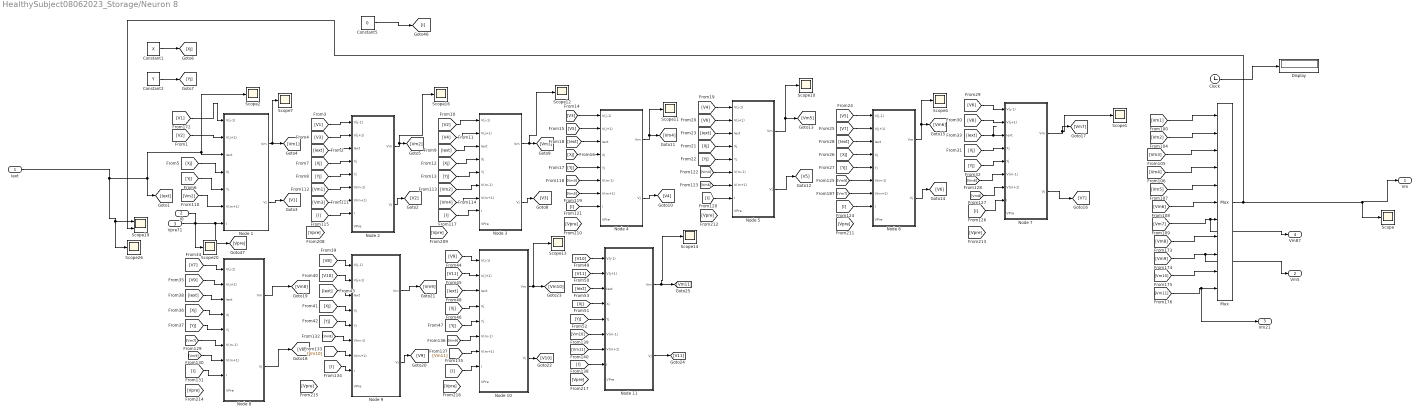
== system HealthySubject08062023_Storage/Neuron 8 ==
  Iext : Inport
  I0 : Inport  Port=2
  Vpre71 : Inport  Port=3
  Clock : Clock
  Constant1 : Constant  Value=X
  Constant2 : Constant  Value=Y
  Constant5 : Constant  Value=0
  Display : Display
  Mux : Mux  Inputs=11
  Node 1 : Subsystem
      mask init:
      | p=1
  Node 10 : Subsystem
      mask init:
      | p=10
  Node 11 : Subsystem
      mask init:
      | p=11
  Node 2 : Subsystem
      mask init:
      | p=2
  Node 3 : Subsystem
      mask init:
      | p=3
  Node 4 : Subsystem
      mask init:
      | p=4
  Node 5 : Subsystem
      mask init:
      | p=5
  Node 6 : Subsystem
      mask init:
      | p=6
  Node 7 : Subsystem
      mask init:
      | p=7
  Node 8 : Subsystem
      mask init:
      | p=8
  Node 9 : Subsystem
      mask init:
      | p=9
  Scope{,1..2,4,7,10..14,16,20,26} (13 alike) : Scope
  Scope19 : Scope  NumInputPorts=2
  Vm : Outport  VectorParamsAs1DForOutWhenUnconnected=off
  Vm5 : Outport  Port=2  VectorParamsAs1DForOutWhenUnconnected=off
  Vm21 : Outport  Port=3  VectorParamsAs1DForOutWhenUnconnected=off
  Vm87 : Outport  Port=4  VectorParamsAs1DForOutWhenUnconnected=off
  wires:
  [Yj] -> Node 2/5(Yj)
  [Xj] -> Node 1/4(Xj)
  Node 1/1(Vm) -> Scope7/1, [Vm1]
  [V2] -> Node 1/2("V(j+1) ")
  Constant1/1 -> [Xj]
  [Xj] -> Node 3/4(Xj)
  [V1] -> Node 1/1(V(j-1))
  Node 2/2(Vj) -> [V2]
  Constant2/1 -> [Yj]
  Node 1/2(Vj) -> [V1]
  [Yj] -> Node 3/5(Yj)
  [Iext] -> Node 3/3(Iext)
  [V2] -> Node 3/1(V(j-1))
  [V1] -> Node 2/1(V(j-1))
  [V4] -> Node 3/2("V(j+1) ")
  Node 3/2(Vj) -> [V3]
  Node 4/2(Vj) -> [V4]
  [V5] -> Node 4/2("V(j+1) ")
  Node 2/1(Vm) -> Scope16/1, [Vm2]
  [Xj] -> Node 2/4(Xj)
  [Iext] -> Node 2/3(Iext)
  Node 4/1(Vm) -> Scope11/1, [Vm4]
  [V3] -> Node 2/2("V(j+1) ")
  [Yj] -> Node 1/5(Yj)
  [V7] -> Node 8/1(V(j-1))
  [V9] -> Node 10/1(V(j-1))
  Node 11/2(Vj) -> [V11]
  [Xj] -> Node 11/4(Xj)
  [Yj] -> Node 11/5(Yj)
  [Iext] -> Node 7/3(Iext)
  Node 6/2(Vj) -> [V6]
  Node 11/1(Vm) -> Scope14/1, [Vm11]
  [Xj] -> Node 5/4(Xj)
  [Xj] -> Node 9/4(Xj)
  [V8] -> Node 7/2("V(j+1) ")
  [Iext] -> Node 6/3(Iext)
  [Xj] -> Node 6/4(Xj)
  [V10] -> Node 9/2("V(j+1) ")
  [Iext] -> Node 11/3(Iext)
  [V10] -> Node 11/1(V(j-1))
  [Iext] -> Node 9/3(Iext)
  [V11] -> Node 11/2("V(j+1) ")
  [V5] -> Node 6/1(V(j-1))
  [Xj] -> Node 8/4(Xj)
  [Yj] -> Node 10/5(Yj)
  [Iext] -> Node 10/3(Iext)
  [V8] -> Node 9/1(V(j-1))
  [Yj] -> Node 4/5(Yj)
  Node 5/1(Vm) -> Scope10/1, [Vm5]
  [Yj] -> Node 7/5(Yj)
  [V7] -> Node 6/2("V(j+1) ")
  [Iext] -> Node 5/3(Iext)
  [Iext] -> Node 4/3(Iext)
  [Xj] -> Node 4/4(Xj)
  [V11] -> Node 10/2("V(j+1) ")
  [Yj] -> Node 6/5(Yj)
  [V3] -> Node 4/1(V(j-1))
  [Yj] -> Node 5/5(Yj)
  Node 8/2(Vj) -> [V8]
  [Yj] -> Node 9/5(Yj)
  [Xj] -> Node 10/4(Xj)
  [Iext] -> Node 8/3(Iext)
  Node 6/1(Vm) -> Scope4/1, [Vm6]
  [V6] -> Node 7/1(V(j-1))
  [V9] -> Node 8/2("V(j+1) ")
  Node 5/2(Vj) -> [V5]
  [Yj] -> Node 8/5(Yj)
  [Vm3] -> Mux/3
  [Vm1] -> Node 2/6(V(m-1))
  [Vm2] -> Node 3/6(V(m-1))
  Constant5/1 -> [I]
  I0/1 -> Node 1/7("I "), Scope20/1
  [Vm2] -> Mux/2
  [Vm2] -> Node 1/6(V(m+1))
  [Vm3] -> Node 4/6(V(m-1))
  [I] -> Node 2/8("I ")
  [I] -> Node 5/8("I ")
  [Vm4] -> Node 5/6(V(m-1))
  [I] -> Node 6/8("I ")
  [Vm4] -> Mux/4
  [Vm3] -> Node 2/7(V(m+1))
  [I] -> Node 9/8("I ")
  Node 9/1(Vm) -> [Vm9]
  [Vm10] -> Node 11/6(V(m-1))
  Node 8/1(Vm) -> [Vm8]
  [Vm6] -> Node 7/6(V(m-1))
  Node 9/2(Vj) -> [V9]
  [Vm8] -> Node 7/7(V(m+1))
  [Vm10] -> Node 9/7(V(m+1))
  [I] -> Node 7/8("I ")
  [Vm9] -> Node 10/6(V(m-1))
  [Vm5] -> Node 6/6(V(m-1))
  [Vm6] -> Mux/6
  [I] -> Node 10/8("I ")
  [Vm7] -> Vm87/1, Mux/7
  [Vm8] -> Mux/8
  [Vm9] -> Vm5/1, Mux/9
  [Vm5] -> Mux/5
  [Vm10] -> Mux/10
  [Vm11] -> Vm21/1, Mux/11
  [Vm9] -> Node 8/7(V(m+1))
  Node 10/1(Vm) -> Scope13/1, [Vm10]
  [Vm7] -> Node 8/6(V(m-1))
  Node 10/2(Vj) -> [V10]
  [Vm8] -> Node 9/6(V(m-1))
  [I] -> Node 8/8("I ")
  Node 7/2(Vj) -> [V7]
  [Vm11] -> Node 10/7(V(m+1))
  [I] -> Node 11/8("I ")
  [Vm11] -> Node 11/7(V(m+1))
  Node 3/1(Vm) -> Scope12/1, [Vm3]
  Mux/1 -> Vm/1, Scope/1, Scope19/2
  [Vm5] -> Node 4/7(V(m+1))
  [Vm6] -> Node 5/7(V(m+1))
  Clock/1 -> Display/1
  Iext/1 -> Scope26/1, Scope19/1, Scope2/1, Node 1/3(Iext), [Iext]
  Node 7/1(Vm) -> [Vm7], Scope1/1
  [Vm7] -> Node 6/7(V(m+1))
  [I] -> Node 4/8("I ")
  Vpre71/1 -> [Vpre]
  [Vm4] -> Node 3/7(V(m+1))
  [I] -> Node 3/8("I ")
  [V6] -> Node 5/2("V(j+1) ")
  [V4] -> Node 5/1(V(j-1))
  [Xj] -> Node 7/4(Xj)
  ? -> ?
  [Vm1] -> Mux/1

== system HealthySubject08062023_Storage/Neuron 9 ==
  V(j-1) : Inport
  "V(j+1) " : Inport  Port=2
  Iext : Inport  Port=3
  Xj : Inport  Port=4
  Yj : Inport  Port=5
  "I " : Inport  Port=6
  Add : Sum  Inputs=+---++-----
  Add1 : Sum  Inputs=+-+
  Constant : Constant  Value=Gaxial
  Divide : Product  Inputs=**
  Gain : Gain  Gain=1/Cn
  Gain1 : Gain  Gain=2
  Integrator : Integrator  InitialCondition=V0
  Ks : Subsystem
  Lk : Subsystem
  Naf : Subsystem
  Nap : Subsystem
  Scope{,1..3} (4 alike) : Scope
  Selector : Selector  InputPortWidth=1  IndexOptions=Index vector (dialog)  Indices=p  OutputSizes=1
  Selector1 : Selector  InputPortWidth=1  IndexOptions=Index vector (dialog)  Indices=p  OutputSizes=1
  Subsystem : Subsystem
  Vm : Outport  VectorParamsAs1DForOutWhenUnconnected=off
  Vj : Outport  Port=2  VectorParamsAs1DForOutWhenUnconnected=off
  wires:
  Divide/1 -> Scope/1, Add/1
  Ks/1(IKs) -> Add/3
  Naf/1("INaf ") -> Add/2
  Add/1 -> Scope3/1, Gain/1
  Lk/1(ILk) -> Add/4
  Add1/1 -> Divide/2
  Gain/1 -> Integrator/1
  Gain1/1 -> Add1/2
  Subsystem/1(Vj) -> Gain1/1, Vj/1
  V(j-1)/1 -> Add1/1
  "V(j+1) "/1 -> Add1/3
  Xj/1 -> Selector/1
  Iext/1 -> Subsystem/1(Iext)
  Selector/1 -> Subsystem/2(Xj)
  Selector1/1 -> Subsystem/3(Yj)
  Yj/1 -> Selector1/1
  "I "/1 -> Add/5
  Constant/1 -> Divide/1
  Nap/1("INap ") -> Add/7
  ? -> Scope1/1, Add/8
  ? -> Add/10
  ? -> Add/11
  ? -> Add/6
  Integrator/1 -> Vm/1, Nap/1(Vm), Lk/1(Vm), Ks/1(Vm), Naf/1(Vm)

== system HealthySubject08062023_Storage/excitatory Neuron 1 ==
  Iext : Inport
  Xj : Inport  Port=2
  Yj : Inport  Port=3
  "I " : Inport  Port=4
  VPreE7 : Inport  Port=5
  Add : Sum  Inputs=+---++-
  Add1 : Sum  Inputs=+-
  Constant2 : Constant  Value=ENaEx
  Divide : Product  Inputs=**
  Gain : Gain  Gain=1/Cn
  Integrator : Integrator  InitialCondition=V0
  Ks : Subsystem
  Lk : Subsystem
  Naf : Subsystem
  Nap1 : Subsystem
  Scope{1..3,5} (4 alike) : Scope
  Selector : Selector  InputPortWidth=1  IndexOptions=Index vector (dialog)  Indices=p  OutputSizes=1
  Selector1 : Selector  InputPortWidth=1  IndexOptions=Index vector (dialog)  Indices=p  OutputSizes=1
  Subsystem : Subsystem
  Transfer Fcn1 : TransferFcn  Denominator=[TawIExt 1]
  Vm : Outport  VectorParamsAs1DForOutWhenUnconnected=off
  wires:
  Divide/1 -> Add/1
  Ks/1(IKs) -> Add/3
  Naf/1("INaf ") -> Add/2
  Add/1 -> Scope3/1, Gain/1
  Lk/1(ILk) -> Scope5/1, Add/4
  Transfer Fcn1/1 -> Divide/2, Scope1/1
  Gain/1 -> Integrator/1
  Subsystem/1(ku) -> Transfer Fcn1/1
  Xj/1 -> Selector/1
  Iext/1 -> Subsystem/1(Iext)
  Selector/1 -> Subsystem/2(Xj)
  Selector1/1 -> Subsystem/3(Yj)
  Yj/1 -> Selector1/1
  "I "/1 -> Add/5
  Add1/1 -> Divide/1
  Constant2/1 -> Add1/1
  Integrator/1 -> Naf/1(Vm), Add1/2, Ks/1(Vm), Lk/1(Vm), Nap1/1(V), Vm/1
  Nap1/1("ISynE ") -> Add/7
  VPreE7/1 -> Nap1/2(Pre)
